simulink model "mcb_pmsm_foc_hall_f28379d"  (R2023b)
settings: Solver=FixedStepDiscrete  StartTime=0.0  StopTime=inf  RelTol=1e-3  EnableMultiTasking=on
InitFcn:
  | mcb_pmsm_foc_hall_f28379d_data;
model workspace (MAT data in the model file):
  encoderResolution = 2000
  hallOffset = '0.5'
  indexOffset = 850
  polePairs = '4'
undefined symbols (not defined in the file): dataType, Down, GPTRIP1SEL, GPTRIP2SEL, inverter, PI_params, pmsm, PosCtrlSpeedLimit, PU_System, target, Ts, Ts_motor, Ts_simulink, Ts_speed, TZ1, TZ2, Up
libraries: simulink x20, c280xlib x17, mcbcontrolslib x9, c2837xDlib x7, c2802xlib x7, svdschedulerlib x5, slpidlib x3, mcbpositiondecoderlib x3, mcbhdlpositiondecoderlib x1, svdutilitieslib x1, mcbplantlib x1, autolibpmsmexterior x1
(part 4 of 4)

== stateflow chart mcb_pmsm_foc_hall_f28379d/EEPROM_Operation_Function ==
  state EEPROM_SUPER
    state EEPROM_GUARD_FUNCTION_STATE [parallel]
      en,du:
      settings: executionOrder=1
      EEPROM_GUARD_FUNCTION_STATE -> (junction 397)
      (junction 397) -> (junction 546) [order 1] : [All_Parameter_Read == true && ...
          | EEPROM_STATUS == t_EEPROM_STATUS_e.EEPROM_STATUS_NOTBUSY]
      (junction 546) -> (junction 548) [order 1] : [Read_Selection_Mnf_Normal == true]
      (junction 397) -> (junction 399) [order 2]
      (junction 546) -> (junction 550) [order 2] : {All_Parameter_Read = false;
          | EEPROM_RWE = t_EEPROM_RWE_e.EEPROM_READ;
          | EEPROM_STATUS = t_EEPROM_STATUS_e.EEPROM_STATUS_BUSY;
          | }
      (junction 548) -> (junction 552) : {All_Parameter_Read = false;
          | EEPROM_StateMachine = ...
          | t_EEPROM_StateMachine_e.EEPROM_OPERATION_MANUFACTURER_DEVICE_ID_STATE
          | }
      (junction 399) -> (junction 400) [order 1] : [All_Parameter_Erase == true && ...
          | EEPROM_STATUS == t_EEPROM_STATUS_e.EEPROM_STATUS_NOTBUSY]
      (junction 399) -> (junction 401) [order 2]
      (junction 400) -> (junction 405) : {All_Parameter_Erase = false;
          | EEPROM_RWE = t_EEPROM_RWE_e.EEPROM_ERASE;
          | EEPROM_STATUS = t_EEPROM_STATUS_e.EEPROM_STATUS_BUSY;}
      (junction 401) -> (junction 402) [order 1] : [All_Parameter_Write == true && ...
          | EEPROM_STATUS == t_EEPROM_STATUS_e.EEPROM_STATUS_NOTBUSY]
      (junction 401) -> (junction 403) [order 2] : {EEPROM_RWE == ...
          | t_EEPROM_RWE_e.EEPROM_DUMMY;}
      (junction 402) -> (junction 404) : {All_Parameter_Write = false;
          | EEPROM_RWE = t_EEPROM_RWE_e.EEPROM_WRITE;
          | EEPROM_STATUS = t_EEPROM_STATUS_e.EEPROM_STATUS_BUSY;}
      (junction 550) -> (junction 552)
      (junction 552) -> (junction 406)
      (junction 404) -> (junction 403)
      (junction 405) -> (junction 404)
      (junction 406) -> (junction 405)
      (junction 403) -> (junction 407)
    state f1 [function]
      (default) -> (junction 431)
      (junction 431) -> (junction 432) [order 1] : [EEPROM_RWE == t_EEPROM_RWE_e.EEPROM_READ]
      (junction 431) -> (junction 433) [order 2]
      (junction 432) -> (junction 440) : {EEPROM_StateMachine =...
          | t_EEPROM_StateMachine_e.EEPROM_OPERATION_READ_DATA_STATE;}
      (junction 433) -> (junction 434) [order 1] : [EEPROM_RWE == t_EEPROM_RWE_e.EEPROM_WRITE]
      (junction 433) -> (junction 435) [order 2]
      (junction 434) -> (junction 439) : {EEPROM_StateMachine = ...
          | t_EEPROM_StateMachine_e.EEPROM_OPERATION_ERASE_ENABLE_STATE;}
      (junction 435) -> (junction 436) [order 1] : [EEPROM_RWE == t_EEPROM_RWE_e.EEPROM_ERASE]
      (junction 435) -> (junction 445) [order 2]
      (junction 436) -> (junction 438) : {EEPROM_StateMachine = ...
          | t_EEPROM_StateMachine_e.EEPROM_OPERATION_ERASE_ENABLE_STATE;}
      (junction 445) -> (junction 447) [order 1] : [EEPROM_RWE_STATUS == t_EEPROM_RWE_STATUS_e.EEPROM_RWE_STATUS_READED]
      (junction 445) -> (junction 449) [order 2]
      (junction 447) -> (junction 451) : {EEPROM_RWE_STATUS = t_EEPROM_RWE_STATUS_e.EEPROM_RWE_STATUS_DUMMY;
          | EEPROM_STATUS = t_EEPROM_STATUS_e.EEPROM_STATUS_NOTBUSY;
          | EEPROM_READ_DATA_AVAILABLE = 1;
          | }
      (junction 449) -> (junction 451) : {EEPROM_STATUS = t_EEPROM_STATUS_e.EEPROM_STATUS_NOTBUSY;}
      (junction 451) -> (junction 454)
      (junction 454) -> (junction 456)
      (junction 456) -> (junction 437)
      (junction 438) -> (junction 437)
      (junction 439) -> (junction 438)
      (junction 440) -> (junction 439)
      (junction 437) -> (junction 441)
    state EEPROM_CONTROLLER_STATE [parallel]
      en,du:
      settings: executionOrder=2
      EEPROM_CONTROLLER_STATE -> (junction 27)
      (junction 27) -> (junction 28) [order 1] : [EEPROM_StateMachine == t_EEPROM_StateMachine_e.EEPROM_OPERATION_DUMMY_STATE]
      (junction 27) -> (junction 31) [order 2]
      (junction 28) -> (junction 29) : {f1();}
      (junction 29) -> (junction 30)
      (junction 30) -> (junction 34)
      (junction 31) -> (junction 32) [order 1] : [EEPROM_StateMachine == t_EEPROM_StateMachine_e.EEPROM_OPERATION_MANUFACTURER_DEVICE_ID_STATE]
      (junction 31) -> (junction 35) [order 2]
      (junction 32) -> (junction 33) : {EEPROM_StateMachine = ...
          | t_EEPROM_StateMachine_e.EEPROM_OPERATION_DUMMY_STATE;
          | Manufacturer_Device_ID_FunctionCall;}
      (junction 33) -> (junction 34)
      (junction 34) -> (junction 38)
      (junction 35) -> (junction 36) [order 1] : [EEPROM_StateMachine == t_EEPROM_StateMachine_e.EEPROM_OPERATION_WRITE_ENABLE_STATE]
      (junction 35) -> (junction 39) [order 2]
      (junction 36) -> (junction 37) : {f2();}
      (junction 37) -> (junction 38)
      (junction 38) -> (junction 42)
      (junction 39) -> (junction 40) [order 1] : [EEPROM_StateMachine == t_EEPROM_StateMachine_e.EEPROM_OPERATION_ERASE_ENABLE_STATE]
      (junction 39) -> (junction 59) [order 2]
      (junction 40) -> (junction 41) : {f5();}
      (junction 41) -> (junction 42)
      (junction 42) -> (junction 57)
      (junction 59) -> (junction 56) [order 1] : [EEPROM_StateMachine == t_EEPROM_StateMachine_e.EEPROM_OPERATION_PAGE_PROGRAM_STATE]
      (junction 59) -> (junction 71) [order 2]
      (junction 56) -> (junction 58) : {f3();}
      (junction 58) -> (junction 57)
      (junction 57) -> (junction 73)
      (junction 71) -> (junction 69) [order 1] : [EEPROM_StateMachine == t_EEPROM_StateMachine_e.EEPROM_OPERATION_READ_DATA_STATE]
      (junction 71) -> (junction 282) [order 2]
      (junction 69) -> (junction 72) : {f4();}
      (junction 72) -> (junction 73)
      (junction 73) -> (junction 281)
      (junction 282) -> (junction 280) [order 1] : [EEPROM_StateMachine == t_EEPROM_StateMachine_e.EEPROM_OPERATION_SECTOR_ERASE_4KB_STATE]
      (junction 282) -> (junction 269) [order 2]
      (junction 280) -> (junction 283) : {f6();}
      (junction 283) -> (junction 281)
      (junction 281) -> (junction 270)
      (junction 270) -> (junction 269)
      (junction 269) -> (junction 271)
    state f2 [function]
      (default) -> (junction 488)
      (junction 488) -> (junction 489) [order 1] : [EEPROM_RWE == t_EEPROM_RWE_e.EEPROM_WRITE]
      (junction 488) -> (junction 490) [order 2]
      (junction 489) -> (junction 491) : {EEPROM_StateMachine = ...
          | t_EEPROM_StateMachine_e.EEPROM_OPERATION_PAGE_PROGRAM_STATE;}
      (junction 491) -> (junction 490)
      (junction 490) -> (junction 492) : {Write_Enable_FunctionCall;}
    state f3 [function]
      (default) -> (junction 495)
      (junction 495) -> (junction 497) : {EEPROM_RWE = t_EEPROM_RWE_e.EEPROM_READ;
          | EEPROM_StateMachine = ...
          | t_EEPROM_StateMachine_e.EEPROM_OPERATION_READ_DATA_STATE;
          | Page_Program_FunctionCall;}
    state f4 [function]
      (default) -> (junction 511)
      (junction 511) -> (junction 512) [order 1] : [EEPROM_RWE == t_EEPROM_RWE_e.EEPROM_WRITE]
      (junction 511) -> (junction 513) [order 2]
      (junction 512) -> (junction 517) : {EEPROM_StateMachine = ...
          | t_EEPROM_StateMachine_e.EEPROM_OPERATION_ERASE_ENABLE_STATE;}
      (junction 513) -> (junction 514) [order 1] : [EEPROM_RWE == t_EEPROM_RWE_e.EEPROM_READ]
      (junction 513) -> (junction 515) [order 2]
      (junction 514) -> (junction 516) : {EEPROM_StateMachine = t_EEPROM_StateMachine_e.EEPROM_OPERATION_DUMMY_STATE;...
          | EEPROM_RWE = t_EEPROM_RWE_e.EEPROM_DUMMY;...
          | EEPROM_RWE_STATUS = t_EEPROM_RWE_STATUS_e.EEPROM_RWE_STATUS_READED;}
      (junction 516) -> (junction 515)
      (junction 517) -> (junction 516)
      (junction 515) -> (junction 518) : {Read_Data_FunctionCall;}
    state f5 [function]
      (default) -> (junction 524)
      (junction 524) -> (junction 522) : {EEPROM_StateMachine = ...
          | t_EEPROM_StateMachine_e.EEPROM_OPERATION_SECTOR_ERASE_4KB_STATE;
          | Write_Enable_FunctionCall;}
    state f6 [function]
      (default) -> (junction 536)
      (junction 536) -> (junction 537) [order 1] : [EEPROM_RWE == t_EEPROM_RWE_e.EEPROM_WRITE]
      (junction 536) -> (junction 538) [order 2]
      (junction 537) -> (junction 542) : {EEPROM_StateMachine = ...
          | t_EEPROM_StateMachine_e.EEPROM_OPERATION_WRITE_ENABLE_STATE;}
      (junction 538) -> (junction 539) [order 1] : [EEPROM_RWE == t_EEPROM_RWE_e.EEPROM_ERASE]
      (junction 538) -> (junction 540) [order 2]
      (junction 539) -> (junction 541) : {EEPROM_StateMachine = t_EEPROM_StateMachine_e.EEPROM_OPERATION_DUMMY_STATE;...
          | EEPROM_RWE = t_EEPROM_RWE_e.EEPROM_DUMMY;}
      (junction 541) -> (junction 540)
      (junction 542) -> (junction 541)
      (junction 540) -> (junction 543) : {Sector_Erase_4KB_FunctionCall;}
  (default) -> EEPROM_SUPER
  data: EEPROM_StateMachine data_store_memory =t_EEPROM_StateMachine_e.EEPROM_OPERATION_DUMMY_STATE; EEPROM_RWE data_store_memory =t_EEPROM_RWE_e.EEPROM_DUMMY; All_Parameter_Read data_store_memory size=1; All_Parameter_Write data_store_memory size=1; All_Parameter_Erase data_store_memory size=1; EEPROM_STATUS data_store_memory =t_EEPROM_STATUS_e.EEPROM_STATUS_NOTBUSY; EEPROM_RWE_STATUS data_store_memory =t_EEPROM_RWE_STATUS_e.EEPROM_RWE_STATUS_DUMMY; Read_Selection_Mnf_Normal input boolean; EEPROM_READ_DATA_AVAILABLE data_store_memory
  events: Manufacturer_Device_ID_FunctionCall output FUNCTION_CALL_EVENT; Write_Enable_FunctionCall output FUNCTION_CALL_EVENT; Page_Program_FunctionCall output FUNCTION_CALL_EVENT; Read_Data_FunctionCall output FUNCTION_CALL_EVENT; Sector_Erase_4KB_FunctionCall output FUNCTION_CALL_EVENT

== stateflow chart mcb_pmsm_foc_hall_f28379d/ID-READ-CALL/Chart ==
  (default) -> (junction 4) : {count = count + 0.5;}
  (junction 4) -> (junction 8) [order 2] : {output = true;}
  (junction 4) -> (junction 8) [order 1] : [count == 1]{count = 0;output = false;}
  data: output output boolean; count local single =0

== stateflow chart mcb_pmsm_foc_hall_f28379d/ENABLE-CALL/Chart ==
  (default) -> (junction 4) : {count = count + 0.5;}
  (junction 4) -> (junction 8) [order 2] : {output = true;}
  (junction 4) -> (junction 8) [order 1] : [count == 1]{count = 0;output = false;}
  data: output output boolean; count local single =0

== stateflow chart mcb_pmsm_foc_hall_f28379d/WRITE-CALL/Chart ==
  (default) -> (junction 4) : {count = count + 0.5;}
  (junction 4) -> (junction 8) [order 2] : {output = true;}
  (junction 4) -> (junction 8) [order 1] : [count == 1]{count = 0;output = false;}
  data: output output boolean; count local single =0

== stateflow chart mcb_pmsm_foc_hall_f28379d/READ-CALL/Chart ==
  (default) -> (junction 4) : {count = count + 0.5;}
  (junction 4) -> (junction 8) [order 2] : {output = true;}
  (junction 4) -> (junction 8) [order 1] : [count == 1]{count = 0;output = false;}
  data: output output boolean; count local single =0

== stateflow chart mcb_pmsm_foc_hall_f28379d/ERASE-CALL/Chart ==
  (default) -> (junction 4) : {count = count + 0.5;}
  (junction 4) -> (junction 8) [order 2] : {output = true;}
  (junction 4) -> (junction 8) [order 1] : [count == 1]{count = 0;output = false;}
  data: output output boolean; count local single =0

== stateflow chart mcb_pmsm_foc_hall_f28379d/Current Control/Control_System/Chart1 ==
  (default) -> (junction 1)
  (junction 1) -> (junction 11) [order 1] : [mode ==1]
  (junction 1) -> (junction 3) [order 2]
  (junction 11) -> (junction 25) : {Auto_nMan_currentRef= false;
      |  Auto_nMan_pos_fdbck= 2;}
  (junction 3) -> (junction 13) [order 1] : [mode==2]
  (junction 3) -> (junction 14) [order 2]
  (junction 13) -> (junction 23) : {Auto_nMan_currentRef= false;
      |  Auto_nMan_pos_fdbck= 3;}
  (junction 14) -> (junction 16) [order 1] : [mode==3]
  (junction 14) -> (junction 19) [order 2]
  (junction 16) -> (junction 21) : {Auto_nMan_currentRef= true;
      |  Auto_nMan_pos_fdbck= 1;
      | offsetReadEnable=true;}
  (junction 21) -> (junction 19)
  (junction 23) -> (junction 21)
  (junction 25) -> (junction 23)
  data: mode input uint16; Auto_nMan_currentRef data_store_memory; Auto_nMan_pos_fdbck data_store_memory; offsetReadEnable output boolean =false

== stateflow chart mcb_pmsm_foc_hall_f28379d/Current Control/Control_System/Direction_Finder_Algorithm/directionFinder ==
  (default) -> (junction 11)
  (junction 11) -> (junction 13) [order 2] : {flag =1;}
  (junction 13) -> (junction 15)
  (junction 11) -> (junction 2) [order 1] : [(flag ==1) && (prevPos ~= Position) ]
  (junction 2) -> (junction 4) : {absDiff = abs(Position-prevPos);}
  (junction 4) -> (junction 19) [order 1] : [absDiff>180]
  (junction 4) -> (junction 25) [order 2]
  (junction 19) -> (junction 33)
  (junction 25) -> (junction 27) [order 1] : [prevPos > Position]
  (junction 25) -> (junction 29) [order 2] : {direction = 1}
  (junction 27) -> (junction 31) : {direction=2}
  (junction 15) -> (junction 29)
  (junction 31) -> (junction 29)
  (junction 33) -> (junction 31)
  (junction 29) -> (junction 38) : {prevPos = Position;}
  data: Position input single; prevPos local single =0; absDiff local single =0; flag local single =0; direction output uint16 =0

== stateflow chart mcb_pmsm_foc_hall_f28379d/Current Control/Control_System/Direction_Finder_Algorithm/deBounce ==
  (default) -> (junction 2)
  (junction 2) -> (junction 21) [order 2]
  (junction 21) -> (junction 23)
  (junction 2) -> (junction 4) [order 1] : [input ~=0 ]
  (junction 4) -> (junction 13) [order 2]
  (junction 13) -> (junction 15) : {cnt = 0;}
  (junction 4) -> (junction 6) [order 1] : [prevValue == input]{cnt = cnt + 1}
  (junction 6) -> (junction 28) [order 2]
  (junction 28) -> (junction 30)
  (junction 6) -> (junction 18) [order 1] : [cnt>5]{Output =input }
  (junction 23) -> (junction 15)
  (junction 15) -> (junction 30)
  (junction 30) -> (junction 18)
  (junction 18) -> (junction 26) : {prevValue = input}
  data: input input uint16; prevValue local uint16 =0; cnt local single =0; Output output uint16 =0

== stateflow chart mcb_pmsm_foc_hall_f28379d/Current Control/Control_System/Sensor_Offset_Algorithm ==
  state Reset
    offsetAngle = 360.0 /  7.0;
  state Init1
    cnt = cnt+1;
    totalPosisiton = totalPosisiton + position;
  state calculation
    entry:
    cnt =0;
    avPosition = totalPosisiton/10.0;
    during:
    avPosition-=offsetAngle;
  state calculationTwo
    offset = -avPosition;
  (default) -> Reset
  Init1 -> calculation : [cnt ==10]
  Reset -> (junction 48) : [enable == 1]
  (junction 48) -> Init1 : after(2,sec)
  calculation -> calculationTwo : [avPosition<=0]
  data: offsetAngle local single; cnt local single; position input single; totalPosisiton local single; avPosition local single; offset output single; enable input boolean

== stateflow chart mcb_pmsm_foc_hall_f28379d/Main_Algorithm1 ==
  state Main_Algorithm
    state Application_State
      state Flash_Read_State
        en,du:
        if(EEPROM_READ_DATA_AVAILABLE == 0)
        All_Parameter_Read = true;
        else
        EEPROM_READ_DATA_AVAILABLE = 0;
        All_Parameter_Read = false;
        if(motor_direction == 1 || motor_direction == 2)
        send(state_end,Application_State);
        else
        send(state_next,Application_State);
        end
        end
      state Motor_Dir_State
        en,du:
        CL_Op_Mode = 1;
        Enable = true;
      state Position_Offset_State
        en,du:
        CL_Op_Mode = 2;
        Enable = true;
      state Flash_Write_State
        en,du:
        All_Parameter_Write = true;
      state App_Run_State
        en,du:
        CL_Op_Mode = 3;
        Enable = false;
      (junction 59) -> (junction 61)
      Flash_Read_State -> (junction 59) [order 2] : [flag==5]
      (junction 61) -> App_Run_State
      (default) -> Flash_Read_State
      Position_Offset_State -> Flash_Write_State : [flag==3]
      Flash_Write_State -> App_Run_State
      Flash_Read_State -> Motor_Dir_State [order 1] : [flag==1]
      Motor_Dir_State -> Position_Offset_State : [flag==2]
    state Motion_Control_State
      state Idle_State
        Enable = false;
      state CloseLoop_State
        en:
        Enable = true;
      (default) -> Idle_State
      Idle_State -> CloseLoop_State : [( Start_Command == true ...
          | && ...
          | CL_Op_Mode == 3 ) || flag==4]
      CloseLoop_State -> Idle_State : [Stop_Command == true]
          | {Enable = false;}
    (default) -> Application_State
    App_Run_State -> (junction 78)
    (junction 78) -> Motion_Control_State
  (default) -> Main_Algorithm
  data: All_Parameter_Read data_store_memory; All_Parameter_Write data_store_memory; EEPROM_READ_DATA_AVAILABLE data_store_memory; motor_direction data_store_memory; Stop_Command data_store_memory; Start_Command data_store_memory; position_offset data_store_memory; CL_Op_Mode data_store_memory; Enable data_store_memory; flag input uint16 =0
  events: state_end local FUNCTION_CALL_EVENT; state_next local FUNCTION_CALL_EVENT
